simulink model "controller"  (R2023b)
settings: Solver=VariableStepDiscrete  StartTime=0.0  StopTime=10.0  FixedStep=Ts  RelTol=1e-3  EnableMultiTasking=on
undefined symbols (not defined in the file): digital_range, direction_range, duty_range, normalized_range, Ts, uint_range_10bit
libraries: simulink x1
settings Model: Creator=jrivitus  LastModifiedBy=student
settings SolverCC: MaxConsecutiveZCs=25  AlgebraicLoopSolver=TrustRegion
settings DataIOCC: DSMLogging=off  ReturnWorkspaceOutputs=off
settings OptimizationCC: DefaultParameterBehavior=Inlined  ExpressionDepthLimit=2147483647  InitFltsAndDblsToZero=on  LifeSpan=1  EfficientTunableParamExpr=on
settings DebuggingCC: UnderspecifiedInitializationDetection=Classic  MergeDetectMultiDrivingBlocksExec=none  ParameterPrecisionLossMsg=none  FcnCallInpInsideContextMsg=warning  UnconnectedInputMsg=warning  UnconnectedOutputMsg=warning  UnconnectedLineMsg=warning  AllowSymbolicDim=off  StateNameClashWarn=warning  PregeneratedLibrarySubsystemCodeDiagnostic=none  SFUnexpectedBacktrackingDiag=warning  SFNoUnconditionalDefaultTransitionDiag=warning  SFExecutionAtInitializationDiag=none  ArithmeticOperatorsInVariantConditions=warning
settings HardwareCC: ProdLongLongMode=on
settings ModelReferenceCC: UpdateModelReferenceTargets=IfOutOfDate  EnableRefExpFcnMdlSchedulingChecks=on  PropagateSignalLabelsOutOfModel=off
settings SFSimCC: SimUseLocalCustomCode=off  MATLABDynamicMemAlloc=off
settings RTWCC: Description=Embedded Coder  SystemTargetFile=ert.tlc  TemplateMakefile=ert_default_tmf  RTWUseLocalCustomCode=off  DLArmComputeVersion=19.05
settings CodeAppCC: IgnoreCustomStorageClasses=off  StateflowObjectComments=on
settings ERTTargetCC: MultiwordLength=2048  GenerateSampleERTMain=on  InlinedParameterPlacement=NonHierarchical  ERTCustomFileTemplate=example_file_process.tlc  ConvertIfToSwitch=off  SuppressUnreachableDefaultCases=off
settings ConfigComp: CovMetricSettings=dcmwe  CovHTMLOptions=-sRT=1 -sVT=0 -aTS=1 -bRG=1 -bTC=1 -hTR=0 -nFC=0 -nFD=1 -scm=1 -bcm=1 -xEv=0 -xEM=0  CovSaveCumulativeToWorkspaceVar=on  CovExternalEMLEnable=off  CovSFcnEnable=off  DVTestSuiteOptimization=CombinedObjectives (Nonlinear Extended)  DVIgnoreExistTestSatisfied=off

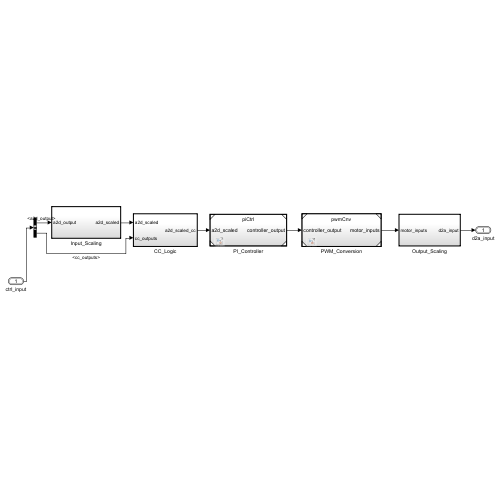
[thumbnail: Simulink's stored preview of the top-level diagram]
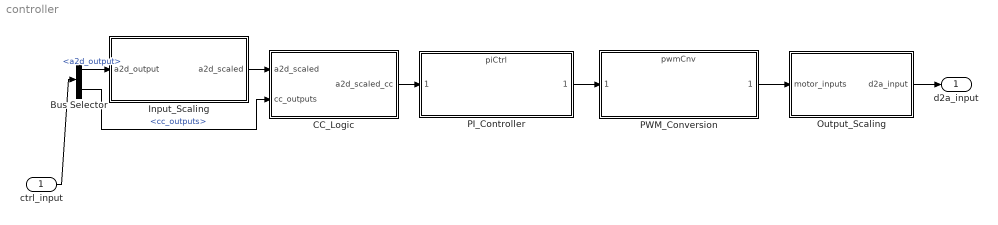
== system controller ==
  ctrl_input : Inport  OutDataTypeStr=Bus: ctrl_input_bus  PortDimensions=1  SampleTime=Ts
  Bus Selector : BusSelector  OutputSignals=a2d_output,cc_outputs
  CC_Logic : Subsystem  TreatAsAtomicUnit=on
  Input_Scaling : Subsystem  RequirementInfo={} %GIDa_d12db97f_5d84_4f01_aa73_1a00163fa707  TreatAsAtomicUnit=on
  Output_Scaling : Subsystem  RequirementInfo={} %GIDa_040f54b5_feae_4999_b3ff_f49e3529df7e  TreatAsAtomicUnit=on
  PI_Controller : ModelReference  ModelNameDialog=piCtrl  SimulationMode=Normal  ModelReferenceVersion=9.0
  PWM_Conversion : ModelReference  ModelNameDialog=pwmCnv  SimulationMode=Normal  ModelReferenceVersion=9.0
  d2a_input : Outport  OutDataTypeStr=Bus: d2a_input_bus  SampleTime=Ts  VectorParamsAs1DForOutWhenUnconnected=off
  wires:
  Output_Scaling/1(d2a_input) -> d2a_input/1
  PWM_Conversion/1 -> Output_Scaling/1(motor_inputs)
  PI_Controller/1 -> PWM_Conversion/1
  Input_Scaling/1(a2d_scaled) -> CC_Logic/1(a2d_scaled)
  Bus Selector/1 -> Input_Scaling/1(a2d_output)  "<a2d_output>"
  ctrl_input/1 -> Bus Selector/1
  CC_Logic/1(a2d_scaled_cc) -> PI_Controller/1
  Bus Selector/2 -> CC_Logic/2(cc_outputs)  "<cc_outputs>"

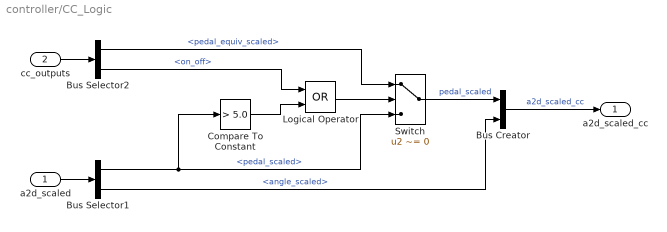
== system controller/CC_Logic ==
  a2d_scaled : Inport  OutDataTypeStr=Bus: a2d_scaled_bus  SampleTime=Ts
  cc_outputs : Inport  Port=2  OutDataTypeStr=Bus: cc_outputs_bus  SampleTime=Ts
  Bus Creator : BusCreator  Inputs=2
  Bus Selector1 : BusSelector  OutputSignals=pedal_scaled,angle_scaled
  Bus Selector2 : BusSelector  OutputSignals=pedal_equiv_scaled,on_off
  Compare To Constant : simulink/Logic and Bit Operations/Compare To Constant  relop=>  const=5.0  OutDataTypeStr=boolean
  Logical Operator : Logic  Operator=OR  AllPortsSameDT=off  OutDataTypeStr=boolean
  Switch : Switch  Criteria=u2 ~= 0  SaturateOnIntegerOverflow=off  InputSameDT=off
      settings: AttributesFormatString="Criteria for passing\\nsignal 1:  %<Criteria>"
  a2d_scaled_cc : Outport  OutDataTypeStr=Bus: a2d_scaled_bus  SampleTime=[0.01,0]  VectorParamsAs1DForOutWhenUnconnected=off
  wires:
  Bus Selector2/2 -> Logical Operator/1  "<on_off>"
  Bus Selector2/1 -> Switch/1  "<pedal_equiv_scaled>"
  Bus Selector1/1 -> Compare To Constant/1, Switch/3  "<pedal_scaled>"
  Switch/1 -> Bus Creator/1  "pedal_scaled"
  cc_outputs/1 -> Bus Selector2/1
  Bus Creator/1 -> a2d_scaled_cc/1  "a2d_scaled_cc"
  Bus Selector1/2 -> Bus Creator/2  "<angle_scaled>"
  a2d_scaled/1 -> Bus Selector1/1
  Logical Operator/1 -> Switch/2
  Compare To Constant/1 -> Logical Operator/2

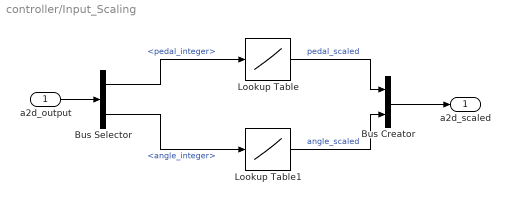
== system controller/Input_Scaling ==
  a2d_output : Inport  OutDataTypeStr=Bus: a2d_output_bus  PortDimensions=1  SampleTime=Ts
  Bus Creator : BusCreator  Inputs=2  OutDataTypeStr=Bus: a2d_scaled_bus
  Bus Selector : BusSelector  OutputSignals=pedal_integer,angle_integer
  Lookup Table : Lookup_n-D  NumberOfTableDimensions=1  BreakpointsForDimension1=uint_range_10bit  Table=normalized_range  ExtrapMethod=Clip  OutDataTypeStr=double
      settings: AttributesFormatString=Output data type: %<OutDataTypeStr>
  Lookup Table1 : Lookup_n-D  NumberOfTableDimensions=1  BreakpointsForDimension1=uint_range_10bit  Table=normalized_range  ExtrapMethod=Clip  OutDataTypeStr=double
      settings: AttributesFormatString=Output data type: %<OutDataTypeStr>
  a2d_scaled : Outport  OutDataTypeStr=Bus: a2d_scaled_bus  SampleTime=Ts  VectorParamsAs1DForOutWhenUnconnected=off
  wires:
  Bus Creator/1 -> a2d_scaled/1
  a2d_output/1 -> Bus Selector/1
  Lookup Table1/1 -> Bus Creator/2  "angle_scaled"
  Bus Selector/2 -> Lookup Table1/1  "<angle_integer>"
  Lookup Table/1 -> Bus Creator/1  "pedal_scaled"
  Bus Selector/1 -> Lookup Table/1  "<pedal_integer>"

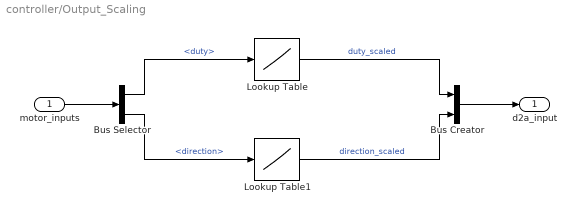
== system controller/Output_Scaling ==
  motor_inputs : Inport  OutDataTypeStr=Bus: motor_inputs_bus  PortDimensions=1  SampleTime=Ts
  Bus Creator : BusCreator  Inputs=2  OutDataTypeStr=Bus: d2a_input_bus
  Bus Selector : BusSelector  OutputSignals=duty,direction
  Lookup Table : Lookup_n-D  NumberOfTableDimensions=1  BreakpointsForDimension1=duty_range  Table=uint_range_10bit  ExtrapMethod=Clip  OutDataTypeStr=uint16
      settings: AttributesFormatString=Output data type: %<OutDataTypeStr>
  Lookup Table1 : Lookup_n-D  NumberOfTableDimensions=1  BreakpointsForDimension1=direction_range  Table=digital_range  ExtrapMethod=Clip  OutDataTypeStr=uint16
      settings: AttributesFormatString=Output data type: %<OutDataTypeStr>
  d2a_input : Outport  OutDataTypeStr=Bus: d2a_input_bus  SampleTime=Ts  VectorParamsAs1DForOutWhenUnconnected=off
  wires:
  motor_inputs/1 -> Bus Selector/1
  Bus Creator/1 -> d2a_input/1
  Lookup Table1/1 -> Bus Creator/2  "direction_scaled"
  Bus Selector/2 -> Lookup Table1/1  "<direction>"
  Bus Selector/1 -> Lookup Table/1  "<duty>"
  Lookup Table/1 -> Bus Creator/1  "duty_scaled"
